simulink model "PIcontrol"  (R2019a)
settings: Solver=VariableStepAuto  StartTime=0.0  StopTime=10.0  MaxStep=1e-3  RelTol=1e-3
values from neighbouring files (symbols this model uses):
  KI = 20    [cruiseControlExample.m]
  KP = 30    [cruiseControlExample.m]
  r = 100*ones(size(t))    [cruiseControlExample.m]
settings Model: Creator=adria  LastModifiedBy=adria

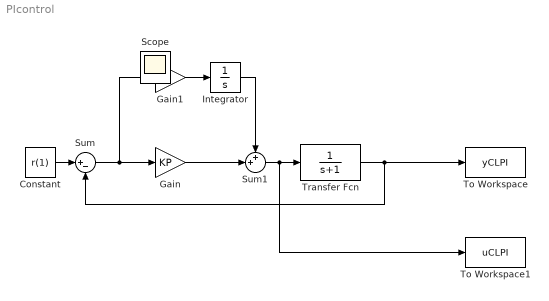
== system PIcontrol ==
  Constant : Constant  Value=r(1)
  Gain : Gain  Gain=KP
  Gain1 : Gain  Gain=KI
  Integrator : Integrator
  Sum : Sum  Inputs=|+-
  Sum1 : Sum  Inputs=++|
  To Workspace : ToWorkspace  VariableName=yCLPI  SaveFormat=Structure With Time  SampleTime=-1
  To Workspace1 : ToWorkspace  VariableName=uCLPI  SaveFormat=Structure With Time  SampleTime=-1
  Transfer Fcn : TransferFcn  Denominator=[1 1]
  Scope : Scope
  wires:
  Sum/1 -> Gain1/1, Gain/1
  Constant/1 -> Sum/1
  Transfer Fcn/1 -> To Workspace/1, Sum/2
  Gain1/1 -> Integrator/1
  Sum1/1 -> To Workspace1/1, Transfer Fcn/1
  Integrator/1 -> Sum1/1
  Gain/1 -> Sum1/2
